simulink model "exp_2"  (R2013b)
settings: Solver=ode3  StartTime=0.0  StopTime=10.0  FixedStep=0.02  RelTol=1e-3
libraries: simulink x2
settings Model: Creator=lenovo  LastModifiedBy=lenovo

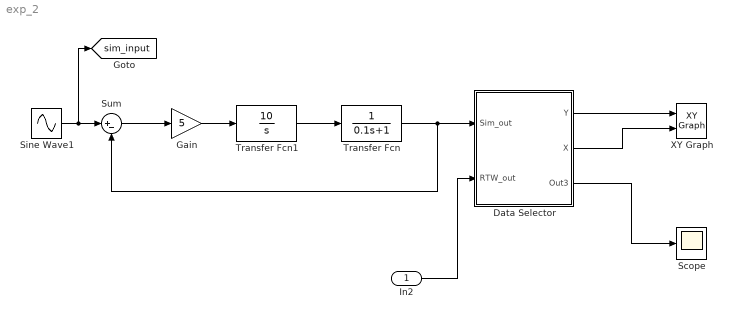
== system exp_2 ==
  In2 : Inport
  "Data Selector " : Subsystem
      mask Display:
      | port_label('output',1,'y')
      | port_label('output',2,'x')
      | port_label('output',3,'Scope')
      | port_label('input',1,'Sim_out')
      | port_label('input',2,'RTW_out')
  Gain : Gain  Gain=5
  Scope : Scope
  Sine Wave1 : Sin  SampleTime=0
  Sum : Sum  Inputs=|+-
  Transfer Fcn : TransferFcn  Denominator=[0.1 1]
  Transfer Fcn1 : TransferFcn  Numerator=[10]  Denominator=[1 0]
  XY Graph : simulink/Sinks/XY Graph  xmin=-1  xmax=1  ymin=-1  ymax=1  st=-1
  tag scope: sim_input=global
  wires:
  Sine Wave1/1 -> [sim_input], Sum/1
  Sum/1 -> Gain/1
  Gain/1 -> Transfer Fcn1/1
  Transfer Fcn1/1 -> Transfer Fcn/1
  Transfer Fcn/1 -> Sum/2, "Data Selector "/1(Sim_out)
  In2/1 -> "Data Selector "/2(RTW_out)
  "Data Selector "/1(Y) -> XY Graph/1
  "Data Selector "/2(X) -> XY Graph/2
  "Data Selector "/3(Out3) -> Scope/1

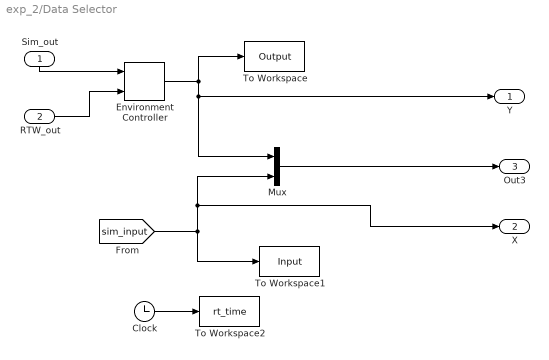
== system exp_2/Data Selector  ==
  Sim_out : Inport
  RTW_out : Inport  Port=2
  Clock : Clock
  Environment Controller : simulink/Signal Routing/Environment Controller
  Mux : Mux  Inputs=2
  To Workspace : ToWorkspace  VariableName=Output  SampleTime=-1  SaveFormat=Timeseries
  To Workspace1 : ToWorkspace  VariableName=Input  SampleTime=-1  SaveFormat=Timeseries
  To Workspace2 : ToWorkspace  VariableName=rt_time  SampleTime=-1  SaveFormat=Timeseries
  Y : Outport
  X : Outport  Port=2
  Out3 : Outport  Port=3
  wires:
  Sim_out/1 -> Environment Controller/1
  [sim_input] -> Mux/2, X/1, To Workspace1/1
  Clock/1 -> To Workspace2/1
  RTW_out/1 -> Environment Controller/2
  Mux/1 -> Out3/1
  Environment Controller/1 -> Mux/1, Y/1, To Workspace/1
